simulink model "mobile_robot_sim"  (R2019a)
settings: Solver=VariableStepAuto  StartTime=0.0  StopTime=5  RelTol=1e-3
values from neighbouring files (symbols this model uses):
  B = 0.188    [calc.m]
  J = 0.0551    [calc.m]
  Kb = 0.062    [calc.m]
  Kp = 1.2*T/(tau*k)    (= 0.284210526316)    [calc.m]    (also in position_control.m = 0.189473684211)
  Kt = 0.062    [calc.m]
  Le = 0.97 * 10^(-3)    (= 0.00097)    [calc.m]
  n = 10    [calc.m]
  Re = 0.56    [calc.m]
  Td = 0    [calc.m]    (also in position_control.m = 0.1)
  Ti = 2*tau    (= 0.4)    [calc.m]    (also in position_control.m = 0.6)
settings Model: Creator=DELL  LastModifiedBy=DELL
settings SolverCC: ZeroCrossAlgorithm=Adaptive
settings DebuggingCC: IgnoredZcDiagnostic=none

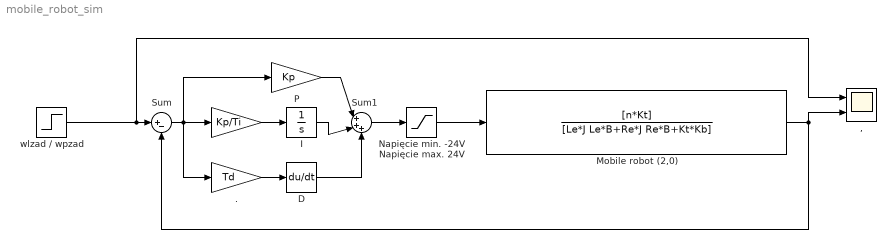
== system mobile_robot_sim ==
  " " : Gain  Gain=Kp/Ti
  ", " : Scope  NumInputPorts=2
  ". " : Gain  Gain=Td
  "D " : Derivative
  "I " : Integrator
  Mobile robot (2,0) : TransferFcn  Numerator=[n*Kt]  Denominator=[Le*J Le*B+Re*J Re*B+Kt*Kb]
  Napięcie min. -24V Napięcie max. 24V : Saturate  UpperLimit=24  LowerLimit=-24
  P : Gain  Gain=Kp
  Sum : Sum  Inputs=|+-
  Sum1 : Sum  Inputs=|+++
  wlzad / wpzad : Step  Time=0  After=25  SampleTime=0
  wires:
  Mobile robot (2,0)/1 -> ", "/2, Sum/2
  Napięcie min. -24V Napięcie max. 24V/1 -> Mobile robot (2,0)/1
  Sum1/1 -> Napięcie min. -24V Napięcie max. 24V/1
  P/1 -> Sum1/1
  Sum/1 -> ". "/1, " "/1, P/1
  " "/1 -> "I "/1
  "I "/1 -> Sum1/2
  wlzad / wpzad/1 -> ", "/1, Sum/1
  "D "/1 -> Sum1/3
  ". "/1 -> "D "/1
